simulink model "partThreeUnicycle"  (R2021b)
settings: Solver=VariableStepAuto  StartTime=0.0  StopTime=10.0  RelTol=1e-3
settings Model: Creator=ericp  LastModifiedBy=ericp

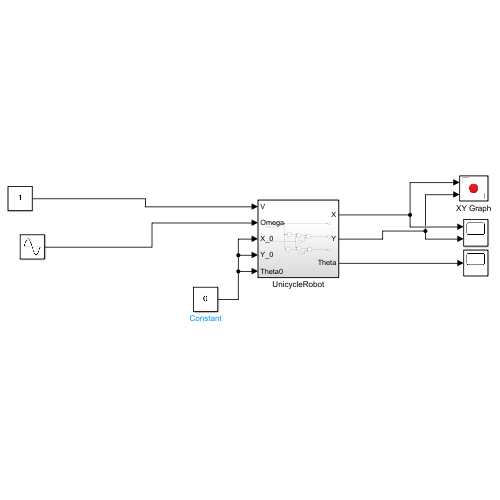
[thumbnail: Simulink's stored preview of the top-level diagram]
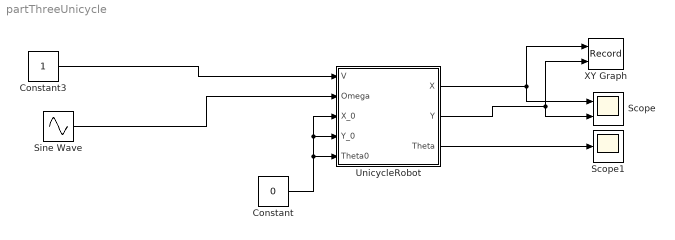
== system partThreeUnicycle ==
  Constant : Constant  Value=0
  Constant3 : Constant
  Scope : Scope  NumInputPorts=2
  Scope1 : Scope
  Sine Wave : Sin  Frequency=100  SampleTime=0
  UnicycleRobot : Subsystem
  XY Graph : Record  FileSettingsInternal="{\"entries\":[{\"content\":{\"excelSettings\":{\"content\":{},\"type\":\"Streamout.ExcelSettings\"}},\"type\":\"Streamout.FileSettingStorage\",\"uuid\":\"6608338a-10d1-4a73-b8fb-88175f70d1b8\"}],\"packageUris\":[\"http://schema.mathworks.com/mf0/streamout_blocks/R2020a\"],\"version\":\"1.0\"}"  Layout=[1 1]  SignalsInternal="{\"entries\":[{\"content\":{\"signals\":[{\"content\":{\"blockPath\":[\"partThreeUnicycle/XY Graph\"],\"channel\":[],\"dimensions\":[1],\"domain\":\"partThreeUnicycle/XY Graph\",\"lineColor\":\"#a2142f\",\"plots\":[1],\"port\":1,\"sid\":[\"\"],\"signalID\":334,\"signalName\":\"UnicycleRobot:2\"},\"type\":\"RecordBlkView.Signal\",\"uuid\":\"55785b7a-f6ec-484f-972e-9221e4c8e800\"},{\"content\":{\"blockPath\":[\"partThreeUnicycle/XY Graph\"],\"channel\":[],\"dimensions\":[1],\"domain\":\"partThreeUnicycle/XY Graph\",\"lineColor\":\"#139fff\",\"plots\":[1],\"port\":2,\"sid\":[\"\"],\"signalID\":338,\"signalName\":\"UnicycleRobot:1\"},\"type\":\"RecordBlkView.Signal\",\"uuid\":\"712038b6-4a6f-49cd-8524-965001537b7a\"}]},\"type\":\"RecordBlkView.InputSignals\",\"uuid\":\"91b7fa18-9a80-4a22-ad22-aab8ab233418\"}],\"packageUris\":[\"http://schema.mathworks.com/mf0/streamout_blocks/R2020a\"],\"version\":\"1.0\"}"  VisualizationBindings="{\"xyplotplugin\":{\"info\":[{\"series\":[{\"bindingParametersList\":[{\"parameter\":\"X-Axis\",\"signalID\":338,\"signalName\":\"UnicycleRobot:1\"},{\"parameter\":\"Y-Axis\",\"signalID\":334,\"signalName\":\"UnicycleRobot:2\"}],\"seriesID\":176}],\"subplotID\":1}]}}"  CompatibilityTag=XY
  wires:
  UnicycleRobot/1(X) -> XY Graph/1, Scope/1
  UnicycleRobot/2(Y) -> XY Graph/2, Scope/2
  UnicycleRobot/3(Theta) -> Scope1/1
  Constant3/1 -> UnicycleRobot/1(V)
  Sine Wave/1 -> UnicycleRobot/2(Omega)
  Constant/1 -> UnicycleRobot/5(Theta0), UnicycleRobot/4(Y_0), UnicycleRobot/3(X_0)

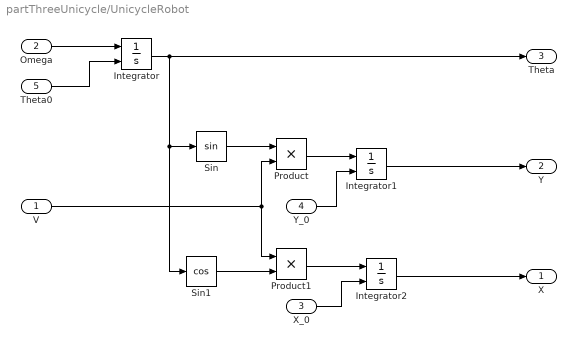
== system partThreeUnicycle/UnicycleRobot ==
  V : Inport
  Omega : Inport  Port=2
  X_0 : Inport  Port=3
  Y_0 : Inport  Port=4
  Theta0 : Inport  Port=5
  Integrator : Integrator  InitialConditionSource=external
  Integrator1 : Integrator  InitialConditionSource=external
  Integrator2 : Integrator  InitialConditionSource=external
  Product : Product
  Product1 : Product
  Sin : Trigonometry
  Sin1 : Trigonometry  Operator=cos
  X : Outport
  Y : Outport  Port=2
  Theta : Outport  Port=3
  wires:
  Sin1/1 -> Product1/2
  V/1 -> Product1/1, Product/2
  Integrator/1 -> Theta/1, Sin1/1, Sin/1
  Integrator2/1 -> X/1
  Sin/1 -> Product/1
  Theta0/1 -> Integrator/2
  Y_0/1 -> Integrator1/2
  Omega/1 -> Integrator/1
  X_0/1 -> Integrator2/2
  Integrator1/1 -> Y/1
  Product1/1 -> Integrator2/1
  Product/1 -> Integrator1/1
